simulink model "NLGantryCrane_bangbang"  (R2017a)
settings: Solver=ode4  StartTime=0.0  StopTime=10  FixedStep=0.01  RelTol=1e-3
values from neighbouring files (symbols this model uses):
  g = 9.81    [Crane_Data.m]    (also in initMIMOgpc.m = mat2cell(gaux,n,m*ones(1,N2)))
  l = 0.5    [Crane_Data.m]
  m1 = 0.5    [Crane_Data.m]
undefined symbols (not defined in the file or in its folder): Amt, Bmt, Cmt
settings Model: Creator=Daniel  LastModifiedBy=Daniel

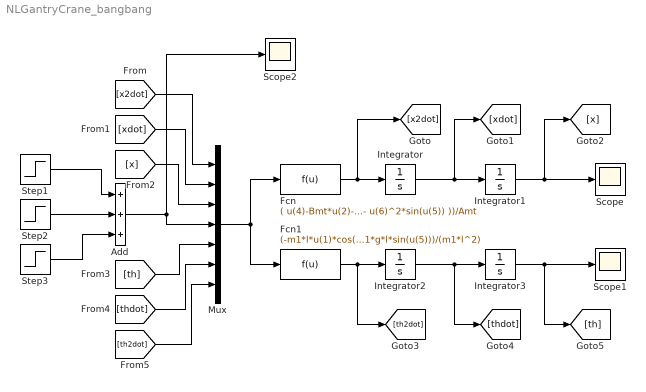
== system NLGantryCrane_bangbang ==
  Add : Sum  Inputs=+++
  Fcn : Fcn  Expr=( u(4)-Bmt*u(2)-Cmt*( u(7)*cos(u(5)) - u(6)^2*sin(u(5)) ))/Amt
  Fcn1 : Fcn  Expr=(-m1*l*u(1)*cos(u(5)) - m1*g*l*sin(u(5)))/(m1*l^2)
  Integrator{,1..3} (4 alike) : Integrator
  Mux : Mux  Inputs=7
  Scope : Scope
  Scope1 : Scope
  Scope2 : Scope
  Step1 : Step  Time=0  After=5  SampleTime=0
  Step2 : Step  After=-10  SampleTime=0
  Step3 : Step  Time=2  After=5  SampleTime=0
  wires:
  Step2/1 -> Add/2
  Step1/1 -> Add/1
  Add/1 -> Mux/4, Scope2/1
  Fcn/1 -> [x2dot], Integrator/1
  Integrator/1 -> [xdot], Integrator1/1
  Integrator1/1 -> [x], Scope/1
  Integrator3/1 -> Scope1/1, [th]
  Integrator2/1 -> Integrator3/1, [thdot]
  Fcn1/1 -> Integrator2/1, [th2dot]
  Mux/1 -> Fcn1/1, Fcn/1
  [th] -> Mux/5
  [x] -> Mux/3
  [thdot] -> Mux/6
  [xdot] -> Mux/2
  [th2dot] -> Mux/7
  [x2dot] -> Mux/1
  Step3/1 -> Add/3
